simulink model "BallHoop"  (Simulink 6.5)
settings: Solver=ode45  StartTime=0.0  StopTime=10  MaxStep=1e-2  RelTol=1e-3
InitFcn:
  | g = 9.81; %gravitational constant
  | 
  |  % showVR = 0; %show VR world
  | %  psi_init = 0; %initial condition
libraries: vrlib x3
CloseFcn:
  | vrclose all;
  | clear figureVR worldVR;
settings Model: Creator=H  LastModifiedBy=Roubalj

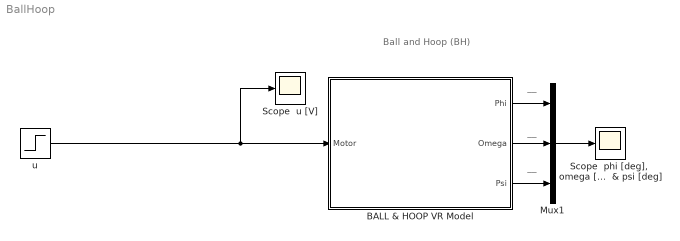
== system BallHoop ==
  note: Ball and Hoop (BH)
  note: __
  note: __
  note: __
  BALL & HOOP VR Model : Subsystem  mask(Ball and Hoop (BH) in laboratory K26){showVR=on, sfcnParam1=0}
      mask prompts: showVR "Show VirtualWorld?"; sfcnParam1 "Initial angle of the ball   psi(0)  [deg]"
      mask help: Ball and Hoop (BH) in laboratory K26 - Virtual Reality
      mask Help:
      | Ball and Hoop in laboratory K26 - Virtual Reality. <br><br>
      | 
      | 
      | This is a virtual model of the Ball and Hoop apparatus in Laboratory of automatic control
      | theory&nbsp;26 (<a href="http://support.dce.felk.cvut.cz/lab26/" target="_blank">http://support.dce.felk.cvut.cz/lab26/</a>),
      | which consists of a&nbsp;DC motor, a&nbsp;hoop and a&nbsp;ball. The&nbsp;hoop angular velocity is controlled
      | by the DC motor controller by the voltage&nbsp;<em>u</em>&nbsp;[V].  A&nbsp;metal ball is placed inside
      | the&nbsp;hoop so that it rolls in a&nbsp;groove on the&nbsp;inner periphery of the&nbsp;hoop.
      | <br><br>
      | 
      | The&nbsp;system input is the&nbsp;voltage of the&nbsp;DC motor&nbsp;<em>u</em>&nbsp;[V].
      | The&nbsp;system outputs are the&nbsp;hoop velocity&nbsp;<em>&omega;</em>&nbsp;[rot/min],
      | the&nbsp;angle of the&nbsp;hoop&nbsp;<em>&phi;</em>&nbsp;[deg] and the&nbsp;angle of
      | the&nbsp;ball&nbsp;<em>&psi;</em>&nbsp;[deg]. More information can be found on the website
      | <a href="http://support.dce.felk.cvut.cz/lab26/" target="_blank">http://support.dce.felk.cvut.cz/lab26/</a>.<br><br>
      | 
      | 
      | In the mask of the model, it can be set:
      | <ul>
      | <li>Initial angle of the ball.</li>
      | </ul><br><br>
      | 
      | 
      | Copyright: 2009, Jiri Machac, Jirka Roubal, Petr Husek.
      mask CallbackString:
      | if strcmp('off',get_param(gcb,'showVR'))
      |     vrclose all;
      | else
      |     if exist('figureVR')==0
      |         figureVR = vrfigure;
      |     end
      |     if exist('worldVR')==0
      |         worldVR = vrworld('BallHoop_VR.WRL');
      |     end
      | 	if isvalid(figureVR)==0
      |         open(worldVR);
      |         figureVR = vrfigure(worldVR,[650 80 550 350]);
      | 	end
      | end|
      mask Display:
      | image(imread('BallHoop_Image.jpg'));
      | port_label ('input',1,'u [V]');
      | port_label ('output',1,'phi [deg]');
      | port_label ('output',2,'omega [rot/min]');
      | port_label ('output',3,'psi [deg]');
  Mux1 : Mux  Inputs=3
  "Scope  phi [deg],  omega [rot/min]  & psi [deg]" : Scope
      settings: TimeRange=10  YMin=-100  YMax=100  SaveName=ty  DataFormat=Array  MaxDataPoints=500000
  Scope  u [V] : Scope
      settings: TimeRange=10  YMin=-10  YMax=10  SaveName=tu  DataFormat=Array  MaxDataPoints=500000
  u : Step  Time=5  Before=-3  After=3  SampleTime=0
  wires:
  BALL & HOOP VR Model/2(Omega) -> Mux1/2
  Mux1/1 -> "Scope  phi [deg],  omega [rot/min]  & psi [deg]"/1
  BALL & HOOP VR Model/3(Psi) -> Mux1/3
  u/1 -> Scope  u [V]/1, BALL & HOOP VR Model/1(Motor)
  BALL & HOOP VR Model/1(Phi) -> Mux1/1

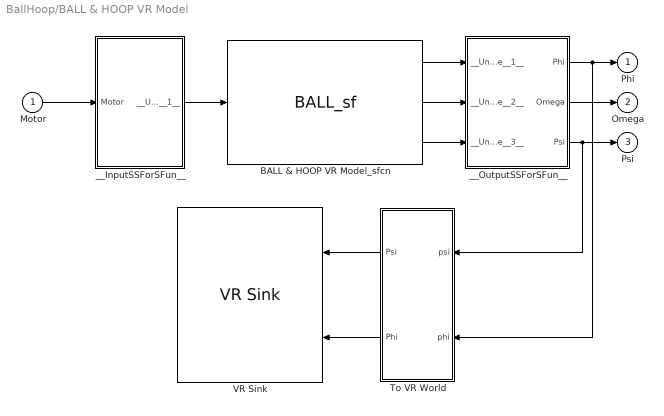
== system BallHoop/BALL & HOOP VR Model ==
  Motor : Inport
  BALL & HOOP VR Model_sfcn : S-Function  FunctionName=BALL_sf  Parameters=sfcnParam1  SFunctionModules=""  mask{rtw_sf_name=BALL_sf, showVar=off, sfcnParam1=sfcnParam1}
      mask prompts: rtw_sf_name "Generated S-function name (model_sf):"; showVar "Show module list"; sfcnParam1 "psi_init:"
      mask help: Real-Time Workshop generated S-function.
      mask init:
      | displist = '';
      | if ~strcmp(get_param(gcb, 'FunctionName'), rtw_sf_name);
      |   set_param(gcb, 'FunctionName', rtw_sf_name);
      | end
      | % Check if we are generating RTW code
      | rtw_mode = false;
      | if strcmpi(get_param(bdroot(gcb),'SimulationStatus'),'Initializing')
      | 	rtw_mode = strcmpi(get_param(bdroot(gcb),'BuildingRTWCode'),'on') && ...
      | 		~strcmpi(get_param(bdroot(gcb),'TargetStyle'),'SimulationTarget');
      | end
      | if showVar || rtw_mode
      | 	if exist('rtwsfunc') == 2 | exist('rtwsfunc') == 6
      | 		tmplist = rtwsfunc(rtw_sf_name,gcb);
      | 		tmplist = ['\nList of Modules:\n', tmplist];
      | 	elseif showVar
      | 		tmplist = '\nList of Modules:\nRTW not licensed\n';
      |  	end
      | end
      | if showVar
      |   displist = tmplist;
      | end
      settings: CopyFcn=set_param(gcb,'LinkStatus','none');
      mask Help: helpview([docroot,'\toolbox\rtw\helptargets.map'],'rtw_Sfunc_target');
      mask Display:
      | port_label('input',1,'Motor');
      | port_label('output',1,'Phi');
      | port_label('output',2,'Omega');
      | port_label('output',3,'Psi');
  To VR World : Subsystem  Orientation=left
  VR Sink : vrlib/VR Sink  Orientation=left  SampleTime=-1  ViewEnable=on  RemoteChange=off  RemoteView=on  FieldsWritten=Ball.rotation.4.1.double#Hoop.rotation.4.1.double  WorldFileName=BallHoop_VR.WRL  AutoView=off  FigureProperties={}
  __InputSSForSFun__ : Subsystem
  __OutputSSForSFun__ : Subsystem
  Phi : Outport  PortDimensions=1  SampleTime=[-1 0]  DataType=double
  Omega : Outport  Port=2  PortDimensions=1  SampleTime=[-1 0]  DataType=double
  Psi : Outport  Port=3  PortDimensions=1  SampleTime=[-1 0]  DataType=double
  wires:
  To VR World/2(Phi) -> VR Sink/2
  To VR World/1(Psi) -> VR Sink/1
  __OutputSSForSFun__/3(Psi) -> To VR World/1(psi), Psi/1
  __OutputSSForSFun__/2(Omega) -> Omega/1
  __OutputSSForSFun__/1(Phi) -> To VR World/2(phi), Phi/1
  BALL & HOOP VR Model_sfcn/3 -> __OutputSSForSFun__/3(__UniqueInportName__3__)
  BALL & HOOP VR Model_sfcn/2 -> __OutputSSForSFun__/2(__UniqueInportName__2__)
  BALL & HOOP VR Model_sfcn/1 -> __OutputSSForSFun__/1(__UniqueInportName__1__)
  __InputSSForSFun__/1(__UniqueOutportName__1__) -> BALL & HOOP VR Model_sfcn/1
  Motor/1 -> __InputSSForSFun__/1(Motor)

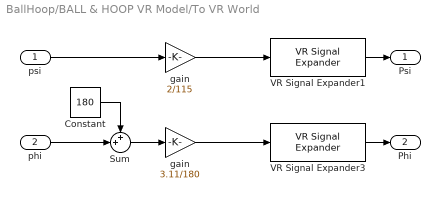
== system BallHoop/BALL & HOOP VR Model/To VR World ==
  psi : Inport
  phi : Inport  Port=2
  Constant : Constant  Value=180  OutDataType=sfix(16)  ConRadixGroup=Use specified scaling  OutScaling=2^0  SampleTime=inf  FramePeriod=inf
  Sum : Sum  Inputs=++|
  VR Signal Expander1 : vrlib/VR Signal Expander  SystemSampleTime=-1  outwidth=4  outidx=[4]
  VR Signal Expander3 : vrlib/VR Signal Expander  SystemSampleTime=-1  outwidth=4  outidx=[4]
  gain : Gain  Gain=2/115
  "gain " : Gain  Gain=3.11/180
  Psi : Outport
  Phi : Outport  Port=2
  wires:
  psi/1 -> gain/1
  VR Signal Expander3/1 -> Phi/1
  VR Signal Expander1/1 -> Psi/1
  phi/1 -> Sum/2
  gain/1 -> VR Signal Expander1/1
  Constant/1 -> Sum/1
  Sum/1 -> "gain "/1
  "gain "/1 -> VR Signal Expander3/1

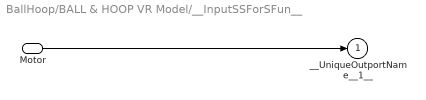
== system BallHoop/BALL & HOOP VR Model/__InputSSForSFun__ ==
  Motor : Inport
  __UniqueOutportName__1__ : Outport
  wires:
  Motor/1 -> __UniqueOutportName__1__/1

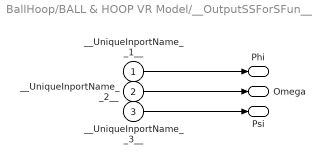
== system BallHoop/BALL & HOOP VR Model/__OutputSSForSFun__ ==
  __UniqueInportName__1__ : Inport
  __UniqueInportName__2__ : Inport  Port=2
  __UniqueInportName__3__ : Inport  Port=3
  Phi : Outport  PortDimensions=1  SampleTime=[-1 0]  DataType=double
  Omega : Outport  Port=2  PortDimensions=1  SampleTime=[-1 0]  DataType=double
  Psi : Outport  Port=3  PortDimensions=1  SampleTime=[-1 0]  DataType=double
  wires:
  __UniqueInportName__3__/1 -> Psi/1
  __UniqueInportName__2__/1 -> Omega/1
  __UniqueInportName__1__/1 -> Phi/1
